simulink model "SecureRoom_ChartEvent"  (R2016a)
settings: Solver=FixedStepDiscrete  StartTime=0.0  StopTime=10.0  RelTol=1e-3
settings Model: Creator=Banna  LastModifiedBy=Banna
settings ConfigSet: Description=Configuration for Code Generation
settings OptimizationCC: DefaultParameterBehavior=Inlined  ActiveStateOutputEnumStorageType=uint8  OptimizeModelRefInitCode=on  LifeSpan=1
settings DebuggingCC: UnderspecifiedInitializationDetection=Classic  MergeDetectMultiDrivingBlocksExec=none
settings ModelReferenceCC: PropagateSignalLabelsOutOfModel=off
settings RTWCC: SystemTargetFile=ert.tlc  GenCodeOnly=on  GenerateMakefile=off  TemplateMakefile=ert_default_tmf  GenerateReport=on  IncludeHyperlinkInReport=on  LaunchReport=on  GenerateTraceInfo=on  GenerateTraceReport=on  GenerateTraceReportSl=on  GenerateTraceReportSf=on  GenerateTraceReportEml=on
settings CodeAppCC: ForceParamTrailComments=on  IgnoreCustomStorageClasses=off  OperatorAnnotations=on  SimulinkDataObjDesc=on  SFDataObjDesc=on  MATLABFcnDesc=on  InsertBlockDesc=on  MATLABSourceComments=on
settings ERTTargetCC: GenerateSampleERTMain=on  SuppressErrorStatus=on  InlinedParameterPlacement=NonHierarchical  ERTCustomFileTemplate=example_file_process.tlc

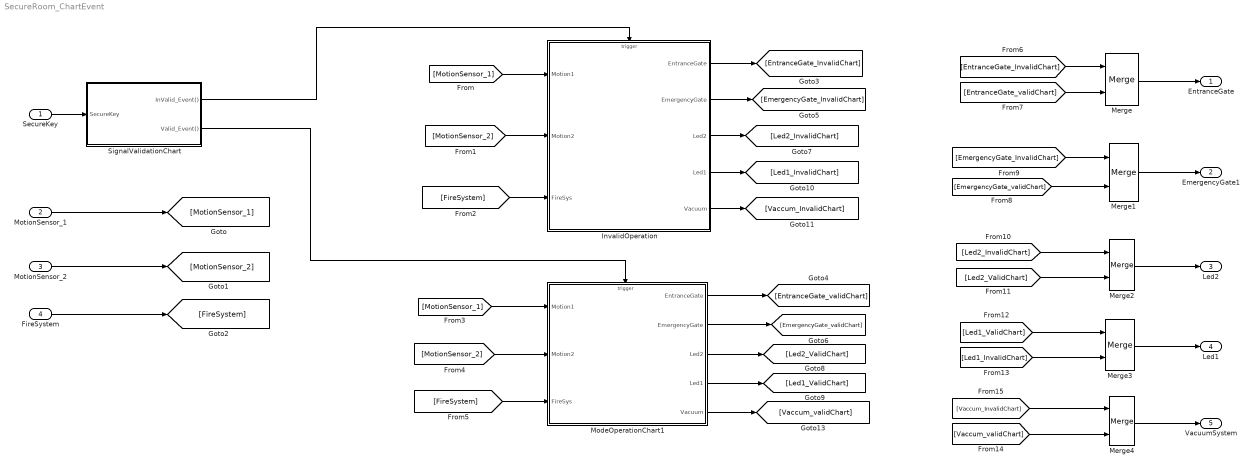
== system SecureRoom_ChartEvent ==
  SecureKey : Inport
  MotionSensor_1 : Inport  Port=2
  MotionSensor_2 : Inport  Port=3
  FireSystem : Inport  Port=4
  InvalidOperation : Stateflow chart  TreatAsAtomicUnit=on
  Merge{,1..4} (5 alike) : Merge
  ModeOperationChart1 : Stateflow chart  TreatAsAtomicUnit=on
  SignalValidationChart : Stateflow chart  TreatAsAtomicUnit=on
  EntranceGate : Outport
  EmergencyGate1 : Outport  Port=2
  Led2 : Outport  Port=3
  "Led1 " : Outport  Port=4
  VacuumSystem : Outport  Port=5
  wires:
  SecureKey/1 -> SignalValidationChart/1(SecureKey)
  SignalValidationChart/1(InValid_Event()) -> InvalidOperation/Trigger
  SignalValidationChart/2(Valid_Event()) -> ModeOperationChart1/Trigger
  MotionSensor_1/1 -> [MotionSensor_1]
  MotionSensor_2/1 -> [MotionSensor_2]
  FireSystem/1 -> [FireSystem]
  [MotionSensor_1] -> InvalidOperation/1(Motion1)
  [MotionSensor_2] -> InvalidOperation/2(Motion2)
  [FireSystem] -> InvalidOperation/3(FireSys)
  [FireSystem] -> ModeOperationChart1/3(FireSys)
  [MotionSensor_2] -> ModeOperationChart1/2(Motion2)
  [MotionSensor_1] -> ModeOperationChart1/1(Motion1)
  Merge/1 -> EntranceGate/1
  Merge1/1 -> EmergencyGate1/1
  Merge3/1 -> "Led1 "/1
  Merge2/1 -> Led2/1
  Merge4/1 -> VacuumSystem/1
  InvalidOperation/1(EntranceGate) -> [EntranceGate_InvalidChart]
  [EntranceGate_InvalidChart] -> Merge/1
  ModeOperationChart1/1(EntranceGate) -> [EntranceGate_validChart]
  [EntranceGate_validChart] -> Merge/2
  InvalidOperation/2(EmergencyGate) -> [EmergencyGate_InvalidChart]
  ModeOperationChart1/2(EmergencyGate) -> [EmergencyGate_validChart]
  [EmergencyGate_validChart] -> Merge1/2
  [EmergencyGate_InvalidChart] -> Merge1/1
  InvalidOperation/3(Led2) -> [Led2_InvalidChart]
  ModeOperationChart1/3(Led2) -> [Led2_ValidChart]
  [Led2_InvalidChart] -> Merge2/1
  [Led2_ValidChart] -> Merge2/2
  InvalidOperation/4(Led1) -> [Led1_InvalidChart]
  ModeOperationChart1/4(Led1) -> [Led1_ValidChart]
  InvalidOperation/5(Vacuum) -> [Vaccum_InvalidChart]
  ModeOperationChart1/5(Vacuum) -> [Vaccum_validChart]
  [Led1_ValidChart] -> Merge3/1
  [Led1_InvalidChart] -> Merge3/2
  [Vaccum_validChart] -> Merge4/2
  [Vaccum_InvalidChart] -> Merge4/1

== stateflow chart SecureRoom_ChartEvent/InvalidOperation ==
  state Invalid
    en:
    EntranceGate=0;
    EmergencyGate=0;
    Led1=0;
    Led2=0;
    Vacuum=0;
    du:
    ex:
  (default) -> Invalid
  data: EntranceGate output; EmergencyGate output; Motion1 input; Motion2 input; Led2 output; Led1 output; Vacuum output; EmergencyCounter local uint8; FireSys input
  events: Invalid_EnableEvent input FUNCTION_CALL_EVENT

== stateflow chart SecureRoom_ChartEvent/ModeOperationChart1 ==
  state Room2
    en:
    Led1=0;
    Led2=1;
    Vacuum=0;
    EntranceGate=1;
    EmergencyGate=1;
    du:
    ex:
  state Room1
    en:
    Led1=1;
    Led2=0;
    Vacuum=0;
    EntranceGate=1;
    EmergencyGate=1;
    du:
    ex:
  state Emergency
    en:
    Led1=1;
    Led2=1;
    Vacuum=1;
    du:
    EmergencyCounter++;
    ex:
  state SystemLocked
    en:
    EntranceGate=0;
    EmergencyGate=0;
    du:
    ex:
  (default) -> Room1
  Room1 -> Room2 [order 1] : [Motion1==0 && Motion2==1]
  Room2 -> Room1 [order 1] : [Motion1==1 && Motion2==0]
  Room2 -> (junction 73) [order 2]
  Room1 -> (junction 74) [order 2]
  (junction 74) -> Emergency : [FireSys==1]
  (junction 73) -> Emergency : [FireSys==1]
  Emergency -> SystemLocked : [EmergencyCounter==5]
  data: EntranceGate output; EmergencyGate output; Motion1 input; Motion2 input; Led2 output; Led1 output; Vacuum output; EmergencyCounter local uint8; FireSys input
  events: ValidEnable_Event input FUNCTION_CALL_EVENT

== stateflow chart SecureRoom_ChartEvent/SignalValidationChart ==
  note: The added condition of "InvalidCounter<3"
      | to prevent counter increment if it reach value = 3
  (default) -> (junction 67) : /* Check on Key Validity */
  (junction 67) -> (junction 68) [order 1] : /*Check if key is invalid for times less than 3*/
      | [SecureKey==0 && InvalidCounter<3]
  (junction 67) -> (junction 69) [order 2]
  (junction 68) -> (junction 73) : /*Increment the error counter*/
      | {InvalidCounter++;}
  (junction 69) -> (junction 70) [order 1] : /*if the key is valid*/
      | [SecureKey==1 && InvalidCounter<3]
  (junction 69) -> (junction 71) [order 2] : /*Do nothing if the
      | Key is invalid for more than three times
      | , system is locked*/
  (junction 70) -> (junction 72) : /*reset the counter*/
      | {InvalidCounter=0;}
  (junction 72) -> (junction 71)
  (junction 73) -> (junction 72)
  (junction 71) -> (junction 45)
  (junction 45) -> (junction 46) [order 1] : /*Invalid Input for three times*/
      | [InvalidCounter==3]
  (junction 45) -> (junction 47) [order 2]
  (junction 46) -> (junction 54) : /*Report Invalid Signal to the System*/
      | {
      | send(InValid_Event);
      | }
  (junction 47) -> (junction 48) [order 1] : /*Invalid signal for time more than one*/
      | [InvalidCounter>0 && SecureKey==0]
  (junction 48) -> (junction 53) : /*Tempory Signal untill
      | signal became stable*/
      | /*do not trigger any event*/
  (junction 47) -> (junction 49) [order 2]
  (junction 49) -> (junction 50) [order 1] : /*Valid Input*/
      | [InvalidCounter==0]
  (junction 49) -> (junction 51) [order 2] : {/*Do Nothing*/;}
  (junction 50) -> (junction 52) : /*Report Valid Signal*/
      | {send(Valid_Event);}
  (junction 52) -> (junction 51)
  (junction 53) -> (junction 52)
  (junction 54) -> (junction 53)
  (junction 51) -> (junction 55)
  data: InvalidCounter local uint8; SecureKey input
  events: InValid_Event output FUNCTION_CALL_EVENT; Valid_Event output FUNCTION_CALL_EVENT
